simulink model "main"  (R2024a)
settings: Solver=FixedStepDiscrete  StartTime=0.0  StopTime=1030/29900  RelTol=1e-3
settings Model: FPTShortcutValueString='{{},{''BaselineRun'',1,1,1,''BaselineRun'','''',{'':6''},''M'','''','''','''',{'':8''},''M'','''','''','''',{},''M'','''',''''}}'  Creator=Jan Rosa  LastModifiedBy=Jan Rosa
settings HardwareCC: ProdBitPerPointer=32  ProdBitPerSizeT=32  ProdBitPerPtrDiffT=32  ProdLargestAtomicFloat=None  ProdIntDivRoundTo=Undefined  ProdEndianess=Unspecified  ProdWordSize=32  ProdHWDeviceType=ASIC/FPGA->ASIC/FPGA  TargetBitPerPointer=64  TargetBitPerSizeT=64  TargetBitPerPtrDiffT=64  TargetLongLongMode=on  TargetIntDivRoundTo=Zero  TargetEndianess=LittleEndian  TargetWordSize=64  TargetHWDeviceType=Custom Processor->MATLAB Host Computer  ProdEqTarget=off

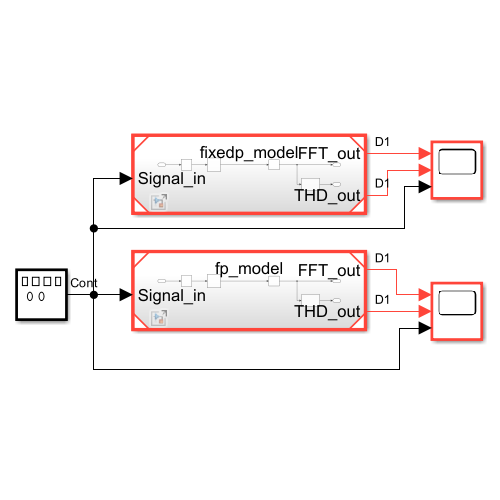
[thumbnail: Simulink's stored preview of the top-level diagram]
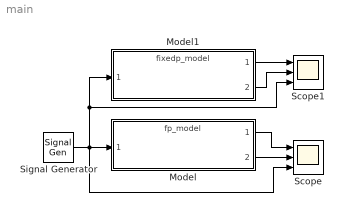
== system main ==
  Model : ModelReference  ModelNameDialog=fp_model.slx  SimulationMode=Normal  ModelReferenceVersion=1.21
  Model1 : ModelReference  ModelNameDialog=fixedp_model.slx  SimulationMode=Normal  ModelReferenceVersion=1.21
  Scope : Scope  NumInputPorts=3
  Scope1 : Scope  NumInputPorts=3
  Signal Generator : SignalGenerator  WaveForm=square  Frequency=230
  wires:
  Signal Generator/1 -> Scope1/3, Model1/1, Scope/3, Model/1
  Model/1 -> Scope/1
  Model/2 -> Scope/2
  Model1/1 -> Scope1/1
  Model1/2 -> Scope1/2
